simulink model "Nugraha_Setya_Ardi"  (R2020b)
settings: Solver=VariableStepAuto  StartTime=0.0  StopTime=0  RelTol=1e-5
libraries: simulink x6, simulink_extras x5, pid_lib x3, sharedtransform x2, aerolibutil x1, vrlib x1
settings Model: Creator=user  LastModifiedBy=nugra

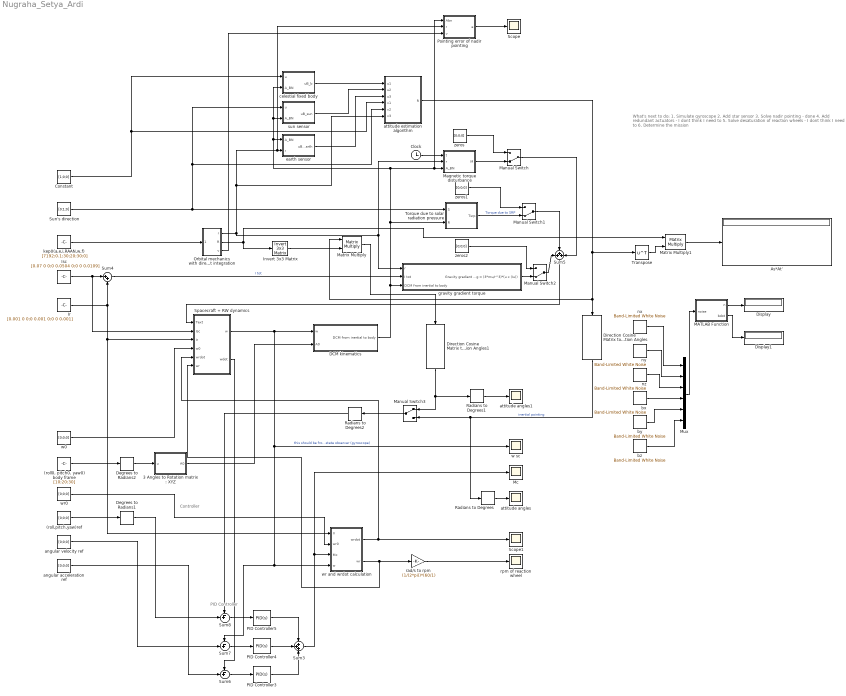
== system Nugraha_Setya_Ardi ==
  note: Controller
  note: PID Controller
  note: What's next to do:
      | 1. Simulate gyroscope
      | 2. Add star sensor
      | 3. Solve nadir pointing - done
      | 4. Add redundant actuators - I dont think I need to
      | 5. Solve desaturation of reaction wheels -  I dont think I need to
      | 6. Determine the mission
  (roll,pitch,yaw)ref : Constant  Value=[0;0;0]  VectorParams1D=off
  "(roll0, pitch0, yaw0) body frame" : Constant  Value=[10;20;30]  VectorParams1D=off
  "3 Angles to Rotation matrix : XYZ" : MATLAB Function  TreatAsAtomicUnit=on
  As*At' : Display
  Clock : Clock
  Constant : Constant  Value=[1;0;0]
  DCM kinematics : Subsystem
  Degrees to Radians1 : simulink_extras/Transformations/Degrees to Radians
  Degrees to Radians2 : simulink_extras/Transformations/Degrees to Radians
  Direction Cosine Matrix to Rotation Angles : sharedtransform/Direction Cosine Matrix to Rotation Angles  rotationOrder=XYZ  aMode=aMode  action=None  tolerance=eps(2)
      settings: SourceProductBaseCode=AE,PW,MT,UV,VE,VP
  Direction Cosine Matrix to Rotation Angles1 : sharedtransform/Direction Cosine Matrix to Rotation Angles  rotationOrder=XYZ  aMode=aMode  action=None  tolerance=eps(2)
      settings: SourceProductBaseCode=AE,PW,MT,UV,VE,VP
  Display : Display
  Display1 : Display
  Invert 3x3 Matrix : aerolibutil/Invert  3x3 Matrix
  Ir : Constant  Value=[0.001 0 0;0 0.001 0;0 0 0.001]  VectorParams1D=off
  Isc : Constant  Value=[0.07 0 0;0 0.0504 0;0 0 0.0109]  VectorParams1D=off
  MATLAB Function : MATLAB Function  TreatAsAtomicUnit=on
  Magnetic torque disturbance : MATLAB Function  TreatAsAtomicUnit=on
  Manual Switch : ManualSwitch  CurrentSetting=0
  Manual Switch1 : ManualSwitch  CurrentSetting=0
  Manual Switch2 : ManualSwitch  CurrentSetting=0
  Manual Switch3 : ManualSwitch
  Matrix Multiply : Product  Multiplication=Matrix(*)
  Matrix Multiply1 : Product  Multiplication=Matrix(*)
  Mc : Scope
  Mux : Mux  Inputs=6
  Orbital mechanics with direct integration : Subsystem
  PID Controller3 : pid_lib/PID Controller  Controller=PID  Form=Parallel  TimeDomain=Continuous-time  UseExternalTs=off  SampleTime=-1  IntegratorMethod=Forward Euler  FilterMethod=Forward Euler  ControllerParametersSource=internal  P=100  I=0  D=0  UseFilter=on  N=100  TunerSelectOption=Transfer Function Based (PID Tuner App)  InitialConditionSource=internal  InitialConditionForIntegrator=0  InitialConditionForFilter=0  DifferentiatorICPrevScaledInput=0  ExternalReset=none  TrackingMode=off  Kt=1  LimitOutput=off  SatLimitsSource=internal  UpperSaturationLimit=inf  LowerSaturationLimit=-inf  LinearizeAsGain=on  AntiWindupMode=none  Kb=1  POutMin=[]  POutMax=[]  IOutMin=[]  IOutMax=[]  DOutMin=[]  DOutMax=[]  NOutMin=[]  NOutMax=[]  SumOutMin=[]  SumOutMax=[]  SaturationOutMin=[]  SaturationOutMax=[]  PParamMin=[]  PParamMax=[]  IParamMin=[]  IParamMax=[]  DParamMin=[]  DParamMax=[]  NParamMin=[]  NParamMax=[]  KbParamMin=[]  KbParamMax=[]  KtParamMin=[]  KtParamMax=[]  KbOutMin=[]  KbOutMax=[]  KtOutMin=[]  KtOutMax=[]  IntegratorOutMin=[]  IntegratorOutMax=[]  FilterOutMin=[]  FilterOutMax=[]  SumI1OutMin=[]  SumI1OutMax=[]  SumI2OutMin=[]  SumI2OutMax=[]  SumI3OutMin=[]  SumI3OutMax=[]  SumI4OutMin=[]  SumI4OutMax=[]  SumDOutMin=[]  SumDOutMax=[]  DifferentiatorOutMin=[]  DifferentiatorOutMax=[]  FilterDiffOutCoefMin=[]  FilterDiffOutCoefMax=[]  ReciprocalOutMin=[]  ReciprocalOutMax=[]  SumDenOutMin=[]  SumDenOutMax=[]  SumNumOutMin=[]  SumNumOutMax=[]  DivideOutMin=[]  DivideOutMax=[]  UdiffTsProdOutMin=[]  UdiffTsProdOutMax=[]  NTsProdOutMin=[]  NTsProdOutMax=[]  UintegralTsProdOutMin=[]  UintegralTsProdOutMax=[]  UngainTsProdOutMin=[]  UngainTsProdOutMax=[]  IntegratorContinuousStateAttributes=''  IntegratorStateMustResolveToSignalObject=off  IntegratorRTWStateStorageClass=Auto  FilterContinuousStateAttributes=''  FilterStateMustResolveToSignalObject=off  FilterRTWStateStorageClass=Auto  ParallelPVariant=InternalParameters  IdealPVariant=Disabled  IVariant=InternalParameters  DVariant=InternalParameters  IntegratorVariant=Continuous  SatVariant=Disabled  AWVariant=Passthrough  PCopyVariant=Disabled  TRVariant=Disabled  FdbkBlocksVariant=Forward  IdealPFdbkVariant=Disabled  SatFdbkVariant=Disabled  DerivativeFilterVariant=ContFilter  NVariant=InternalParameters  NCopyVariant=Disabled  FilterICVariant=InternalICsFilter  IntegratorICVariant=InternalICs  ExternalResetVariant=Disabled  TRSumVariant=Passthrough  SumFdbkVariant=Disabled  SumVariant=Sum_PID  TsampFilterVariant=InternalTs  TsampNgainVariant=Passthrough  TsampIntegralVariant=Passthrough  ExternalSaturationOutDataTypeStr=Inherit: Same as second input
  PID Controller4 : pid_lib/PID Controller  Controller=PID  Form=Parallel  TimeDomain=Continuous-time  UseExternalTs=off  SampleTime=-1  IntegratorMethod=Forward Euler  FilterMethod=Forward Euler  ControllerParametersSource=internal  P=70  I=0  D=0  UseFilter=on  N=100  TunerSelectOption=Transfer Function Based (PID Tuner App)  InitialConditionSource=internal  InitialConditionForIntegrator=0  InitialConditionForFilter=0  DifferentiatorICPrevScaledInput=0  ExternalReset=none  TrackingMode=off  Kt=1  LimitOutput=off  SatLimitsSource=internal  UpperSaturationLimit=inf  LowerSaturationLimit=-inf  LinearizeAsGain=on  AntiWindupMode=none  Kb=1  POutMin=[]  POutMax=[]  IOutMin=[]  IOutMax=[]  DOutMin=[]  DOutMax=[]  NOutMin=[]  NOutMax=[]  SumOutMin=[]  SumOutMax=[]  SaturationOutMin=[]  SaturationOutMax=[]  PParamMin=[]  PParamMax=[]  IParamMin=[]  IParamMax=[]  DParamMin=[]  DParamMax=[]  NParamMin=[]  NParamMax=[]  KbParamMin=[]  KbParamMax=[]  KtParamMin=[]  KtParamMax=[]  KbOutMin=[]  KbOutMax=[]  KtOutMin=[]  KtOutMax=[]  IntegratorOutMin=[]  IntegratorOutMax=[]  FilterOutMin=[]  FilterOutMax=[]  SumI1OutMin=[]  SumI1OutMax=[]  SumI2OutMin=[]  SumI2OutMax=[]  SumI3OutMin=[]  SumI3OutMax=[]  SumI4OutMin=[]  SumI4OutMax=[]  SumDOutMin=[]  SumDOutMax=[]  DifferentiatorOutMin=[]  DifferentiatorOutMax=[]  FilterDiffOutCoefMin=[]  FilterDiffOutCoefMax=[]  ReciprocalOutMin=[]  ReciprocalOutMax=[]  SumDenOutMin=[]  SumDenOutMax=[]  SumNumOutMin=[]  SumNumOutMax=[]  DivideOutMin=[]  DivideOutMax=[]  UdiffTsProdOutMin=[]  UdiffTsProdOutMax=[]  NTsProdOutMin=[]  NTsProdOutMax=[]  UintegralTsProdOutMin=[]  UintegralTsProdOutMax=[]  UngainTsProdOutMin=[]  UngainTsProdOutMax=[]  IntegratorContinuousStateAttributes=''  IntegratorStateMustResolveToSignalObject=off  IntegratorRTWStateStorageClass=Auto  FilterContinuousStateAttributes=''  FilterStateMustResolveToSignalObject=off  FilterRTWStateStorageClass=Auto  ParallelPVariant=InternalParameters  IdealPVariant=Disabled  IVariant=InternalParameters  DVariant=InternalParameters  IntegratorVariant=Continuous  SatVariant=Disabled  AWVariant=Passthrough  PCopyVariant=Disabled  TRVariant=Disabled  FdbkBlocksVariant=Forward  IdealPFdbkVariant=Disabled  SatFdbkVariant=Disabled  DerivativeFilterVariant=ContFilter  NVariant=InternalParameters  NCopyVariant=Disabled  FilterICVariant=InternalICsFilter  IntegratorICVariant=InternalICs  ExternalResetVariant=Disabled  TRSumVariant=Passthrough  SumFdbkVariant=Disabled  SumVariant=Sum_PID  TsampFilterVariant=InternalTs  TsampNgainVariant=Passthrough  TsampIntegralVariant=Passthrough  ExternalSaturationOutDataTypeStr=Inherit: Same as second input
  PID Controller5 : pid_lib/PID Controller  Controller=PID  Form=Parallel  TimeDomain=Continuous-time  UseExternalTs=off  SampleTime=-1  IntegratorMethod=Forward Euler  FilterMethod=Forward Euler  ControllerParametersSource=internal  P=10  I=0  D=0  UseFilter=on  N=100  TunerSelectOption=Transfer Function Based (PID Tuner App)  InitialConditionSource=internal  InitialConditionForIntegrator=0  InitialConditionForFilter=0  DifferentiatorICPrevScaledInput=0  ExternalReset=none  TrackingMode=off  Kt=1  LimitOutput=off  SatLimitsSource=internal  UpperSaturationLimit=inf  LowerSaturationLimit=-inf  LinearizeAsGain=on  AntiWindupMode=none  Kb=1  POutMin=[]  POutMax=[]  IOutMin=[]  IOutMax=[]  DOutMin=[]  DOutMax=[]  NOutMin=[]  NOutMax=[]  SumOutMin=[]  SumOutMax=[]  SaturationOutMin=[]  SaturationOutMax=[]  PParamMin=[]  PParamMax=[]  IParamMin=[]  IParamMax=[]  DParamMin=[]  DParamMax=[]  NParamMin=[]  NParamMax=[]  KbParamMin=[]  KbParamMax=[]  KtParamMin=[]  KtParamMax=[]  KbOutMin=[]  KbOutMax=[]  KtOutMin=[]  KtOutMax=[]  IntegratorOutMin=[]  IntegratorOutMax=[]  FilterOutMin=[]  FilterOutMax=[]  SumI1OutMin=[]  SumI1OutMax=[]  SumI2OutMin=[]  SumI2OutMax=[]  SumI3OutMin=[]  SumI3OutMax=[]  SumI4OutMin=[]  SumI4OutMax=[]  SumDOutMin=[]  SumDOutMax=[]  DifferentiatorOutMin=[]  DifferentiatorOutMax=[]  FilterDiffOutCoefMin=[]  FilterDiffOutCoefMax=[]  ReciprocalOutMin=[]  ReciprocalOutMax=[]  SumDenOutMin=[]  SumDenOutMax=[]  SumNumOutMin=[]  SumNumOutMax=[]  DivideOutMin=[]  DivideOutMax=[]  UdiffTsProdOutMin=[]  UdiffTsProdOutMax=[]  NTsProdOutMin=[]  NTsProdOutMax=[]  UintegralTsProdOutMin=[]  UintegralTsProdOutMax=[]  UngainTsProdOutMin=[]  UngainTsProdOutMax=[]  IntegratorContinuousStateAttributes=''  IntegratorStateMustResolveToSignalObject=off  IntegratorRTWStateStorageClass=Auto  FilterContinuousStateAttributes=''  FilterStateMustResolveToSignalObject=off  FilterRTWStateStorageClass=Auto  ParallelPVariant=InternalParameters  IdealPVariant=Disabled  IVariant=InternalParameters  DVariant=InternalParameters  IntegratorVariant=Continuous  SatVariant=Disabled  AWVariant=Passthrough  PCopyVariant=Disabled  TRVariant=Disabled  FdbkBlocksVariant=Forward  IdealPFdbkVariant=Disabled  SatFdbkVariant=Disabled  DerivativeFilterVariant=ContFilter  NVariant=InternalParameters  NCopyVariant=Disabled  FilterICVariant=InternalICsFilter  IntegratorICVariant=InternalICs  ExternalResetVariant=Disabled  TRSumVariant=Passthrough  SumFdbkVariant=Disabled  SumVariant=Sum_PID  TsampFilterVariant=InternalTs  TsampNgainVariant=Passthrough  TsampIntegralVariant=Passthrough  ExternalSaturationOutDataTypeStr=Inherit: Same as second input
  Pointing error of nadir pointing : MATLAB Function  TreatAsAtomicUnit=on
  Radians to Degrees : simulink_extras/Transformations/Radians to Degrees
  Radians to Degrees1 : simulink_extras/Transformations/Radians to Degrees
  Radians to Degrees2 : simulink_extras/Transformations/Radians to Degrees
  Scope : Scope
  Scope1 : Scope
  Spacecraft + RW dynamics : Subsystem
  Sum3 : Sum  Inputs=+++
  Sum4 : Sum  Inputs=|++
  Sum5 : Sum  Inputs=+++
  Sum6 : Sum  Inputs=-+|
  Sum7 : Sum  Inputs=-+|
  Sum8 : Sum  Inputs=-+|
  Sun's direction : Constant  Value=[0;1;0]
  Torque due to solar radiation pressure : MATLAB Function  TreatAsAtomicUnit=on
  Transpose : Math  Operator=transpose  SaturateOnIntegerOverflow=on
  angular acceleration ref : Constant  Value=[0;0;0]
  angular velocity ref : Constant  Value=[0;0;0]  VectorParams1D=off
  attitude angles : Scope
  attitude angles1 : Scope
  attitude estimation algorithm : MATLAB Function  TreatAsAtomicUnit=on
  bx : simulink/Sources/Band-Limited White Noise  Cov=[0.0001]  Ts=0.001  seed=[236431]
  by : simulink/Sources/Band-Limited White Noise  Cov=[0.0001]  Ts=0.001  seed=[768541]
  bz : simulink/Sources/Band-Limited White Noise  Cov=[0.0001]  Ts=0.001  seed=[287921]
  celestial fixed body : MATLAB Function  TreatAsAtomicUnit=on
  earth sensor : MATLAB Function  TreatAsAtomicUnit=on
  gravity gradient torque : Subsystem
  kep0(a,e,i,RAAN,w,f) : Constant  Value=[7192;0.1;30;20;30;0]  VectorParams1D=off
  nx : simulink/Sources/Band-Limited White Noise  Cov=[0.0001]  Ts=0.01  seed=[23341]
  ny : simulink/Sources/Band-Limited White Noise  Cov=[0.0001]  Ts=0.001  seed=[6341]
  nz : simulink/Sources/Band-Limited White Noise  Cov=[0.0001]  Ts=0.001  seed=[2335671]
  rad/s to rpm : Gain  Gain=(1/(2*pi))*(60/1)
  rpm of reaction wheel : Scope
  sun sensor : MATLAB Function  TreatAsAtomicUnit=on
  w sc : Scope
  w0 : Constant  Value=[0;0;0]
  wr and wrdot calculation : Subsystem
  wr0 : Constant  Value=[0;0;0]
  zeros : Constant  Value=[0;0;0]  VectorParams1D=off
  zeros1 : Constant  Value=[0;0;0]  VectorParams1D=off
  zeros2 : Constant  Value=[0;0;0]  VectorParams1D=off
  wires:
  Isc/1 -> Spacecraft + RW dynamics/2(Isc), Sum4/1
  Ir/1 -> wr and wrdot calculation/1(Ir), Spacecraft + RW dynamics/3(Ir), Sum4/2
  w0/1 -> Spacecraft + RW dynamics/4(w0)
  "(roll0, pitch0, yaw0) body frame"/1 -> Degrees to Radians2/1
  (roll,pitch,yaw)ref/1 -> Degrees to Radians1/1
  angular velocity ref/1 -> Sum7/2
  angular acceleration ref/1 -> Sum6/2
  Degrees to Radians1/1 -> Sum8/2
  Degrees to Radians2/1 -> "3 Angles to Rotation matrix : XYZ"/1(u)
  Torque due to solar radiation pressure/1(Tsrp) -> Manual Switch1/2  "Torque due to SRP"
  Radians to Degrees/1 -> attitude angles/1
  rad/s to rpm/1 -> rpm of reaction wheel/1
  gravity gradient torque/1(Gravity gradient torque Mgg = (3*mu/r^3)*(u x (Iu))) -> Manual Switch2/2
  Sum4/1 -> gravity gradient torque/2(I tot)  "I tot"
  kep0(a,e,i,RAAN,w,f)/1 -> Orbital mechanics with direct integration/1(kep0)
  Sum5/1 -> Spacecraft + RW dynamics/1(Text)
  Spacecraft + RW dynamics/2(wdot) -> Sum6/1
  "3 Angles to Rotation matrix : XYZ"/1(A0) -> DCM kinematics/2(A0)
  wr and wrdot calculation/1(wrdot) -> Spacecraft + RW dynamics/5(wrdot), Scope1/1
  wr and wrdot calculation/2(wr) -> rad/s to rpm/1, Spacecraft + RW dynamics/6(wr)
  wr0/1 -> wr and wrdot calculation/2(wr0)
  Sum6/1 -> PID Controller3/1
  Sum7/1 -> PID Controller4/1
  PID Controller5/1 -> Sum3/1
  PID Controller4/1 -> Sum3/2
  PID Controller3/1 -> Sum3/3
  Sum3/1 -> Mc/1, wr and wrdot calculation/3(Mc)
  Orbital mechanics with direct integration/1(r) -> gravity gradient torque/1(r), Magnetic torque disturbance/2(r), attitude estimation algorithm/6(v3), Pointing error of nadir pointing/2(r), earth sensor/2(r)
  DCM kinematics/1(DCM from inertial to body) -> earth sensor/1(A_BN), celestial fixed body/2(A_BN), sun sensor/2(A_BN), Pointing error of nadir pointing/1(Abn), Magnetic torque disturbance/3(A_BN), Torque due to solar radiation pressure/2(R), gravity gradient torque/3(DCM from inertial to body)
  Clock/1 -> Magnetic torque disturbance/1(t)
  Magnetic torque disturbance/1(M) -> Manual Switch/2
  zeros/1 -> Manual Switch/1
  Manual Switch/1 -> Sum5/3
  zeros1/1 -> Manual Switch1/1
  Manual Switch1/1 -> Sum5/2
  zeros2/1 -> Manual Switch2/1
  Manual Switch2/1 -> Sum5/1
  Sun's direction/1 -> sun sensor/1(u), attitude estimation algorithm/5(v2), Torque due to solar radiation pressure/1(S)
  sun sensor/1(uB_sun) -> attitude estimation algorithm/2(u2)
  earth sensor/1(uB_earth) -> attitude estimation algorithm/3(u3)
  Constant/1 -> celestial fixed body/1(u), attitude estimation algorithm/4(v1)
  celestial fixed body/1(uB_b) -> attitude estimation algorithm/1(u1)
  attitude estimation algorithm/1(R) -> Transpose/1, Matrix Multiply/1, Direction Cosine Matrix to Rotation Angles/1
  Direction Cosine Matrix to Rotation Angles/1 -> Radians to Degrees/1, Manual Switch3/2  "inertial pointing"
  Spacecraft + RW dynamics/1(w) -> Sum7/1, wr and wrdot calculation/4(w), w sc/1, DCM kinematics/1(w)  "this should be from state observer (gyroscope)"
  Orbital mechanics with direct integration/2(R) -> Invert 3x3 Matrix/1, Matrix Multiply1/1
  Sum8/1 -> PID Controller5/1
  Invert 3x3 Matrix/1 -> Matrix Multiply/2
  Matrix Multiply/1 -> Direction Cosine Matrix to Rotation Angles1/1
  Manual Switch3/1 -> Radians to Degrees2/1
  Direction Cosine Matrix to Rotation Angles1/1 -> Radians to Degrees1/1, Manual Switch3/1
  Radians to Degrees1/1 -> attitude angles1/1
  Transpose/1 -> Matrix Multiply1/2
  Matrix Multiply1/1 -> As*At'/1
  Pointing error of nadir pointing/1(e) -> Scope/1
  Orbital mechanics with direct integration/3(v) -> Pointing error of nadir pointing/3(v)
  Radians to Degrees2/1 -> Sum8/1
  MATLAB Function/1(n) -> Display/1
  MATLAB Function/2(bdot) -> Display1/1
  nx/1 -> Mux/1
  ny/1 -> Mux/2
  nz/1 -> Mux/3
  bx/1 -> Mux/4
  by/1 -> Mux/5
  bz/1 -> Mux/6
  Mux/1 -> MATLAB Function/1(noise)

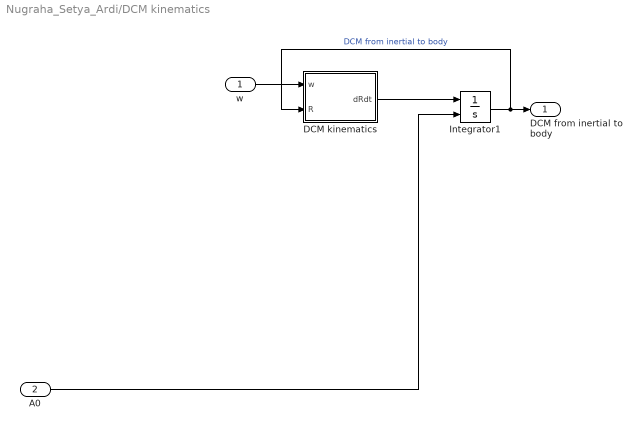
== system Nugraha_Setya_Ardi/DCM kinematics ==
  w : Inport
  A0 : Inport  Port=2
  DCM kinematics : MATLAB Function  TreatAsAtomicUnit=on
  Integrator1 : Integrator  InitialConditionSource=external
  DCM from inertial to body : Outport
  wires:
  DCM kinematics/1(dRdt) -> Integrator1/1
  A0/1 -> Integrator1/2
  Integrator1/1 -> DCM kinematics/2(R), DCM from inertial to body/1  "DCM from inertial to body"
  w/1 -> DCM kinematics/1(w)

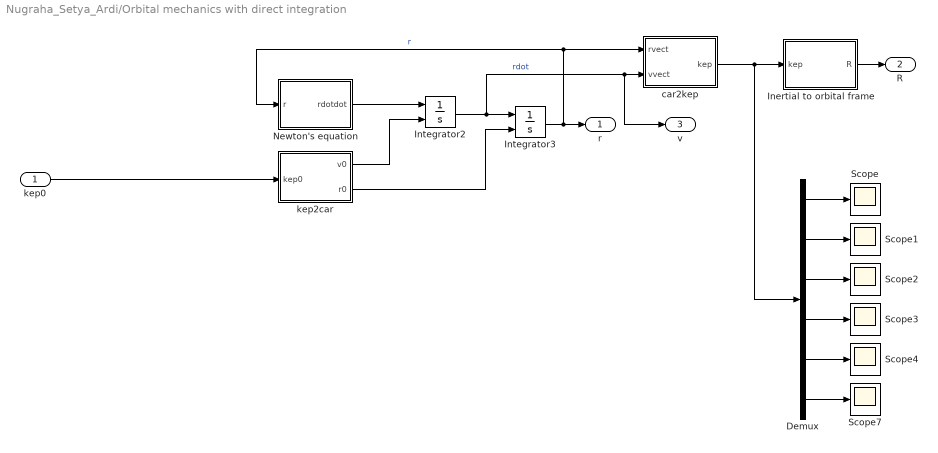
== system Nugraha_Setya_Ardi/Orbital mechanics with direct integration ==
  kep0 : Inport
  Demux : Demux  Outputs=6
  Inertial to orbital frame : MATLAB Function  TreatAsAtomicUnit=on
  Integrator2 : Integrator  InitialConditionSource=external
  Integrator3 : Integrator  InitialConditionSource=external
  Newton's equation : MATLAB Function  TreatAsAtomicUnit=on
  Scope{,1..4,7} (6 alike) : Scope
  car2kep : MATLAB Function  TreatAsAtomicUnit=on
  kep2car : MATLAB Function  TreatAsAtomicUnit=on
  r : Outport
  R : Outport  Port=2
  v : Outport  Port=3
  wires:
  Integrator3/1 -> car2kep/1(rvect), Newton's equation/1(r), r/1  "r"
  Newton's equation/1(rdotdot) -> Integrator2/1
  kep2car/2(r0) -> Integrator3/2
  kep2car/1(v0) -> Integrator2/2
  kep0/1 -> kep2car/1(kep0)
  Integrator2/1 -> v/1, car2kep/2(vvect), Integrator3/1  "rdot"
  car2kep/1(kep) -> Demux/1, Inertial to orbital frame/1(kep)
  Inertial to orbital frame/1(R) -> R/1
  Demux/1 -> Scope/1
  Demux/2 -> Scope1/1
  Demux/3 -> Scope2/1
  Demux/4 -> Scope3/1
  Demux/5 -> Scope4/1
  Demux/6 -> Scope7/1

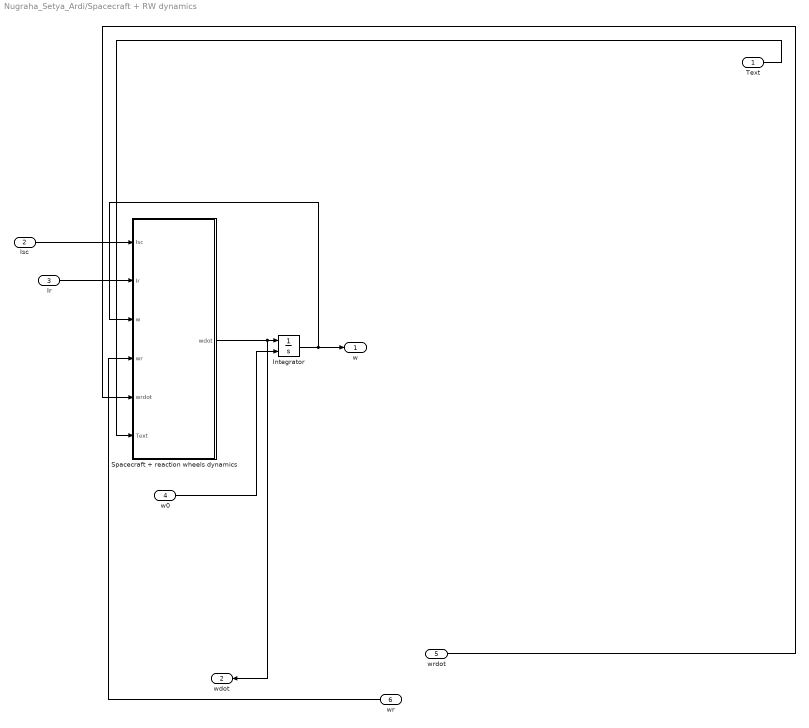
== system Nugraha_Setya_Ardi/Spacecraft + RW dynamics ==
  Text : Inport
  Isc : Inport  Port=2
  Ir : Inport  Port=3
  w0 : Inport  Port=4
  wrdot : Inport  Port=5
  wr : Inport  Port=6
  Integrator : Integrator  InitialConditionSource=external
  Spacecraft + reaction wheels dynamics : MATLAB Function  TreatAsAtomicUnit=on
  w : Outport
  wdot : Outport  Port=2
  wires:
  Text/1 -> Spacecraft + reaction wheels dynamics/6(Text)
  w0/1 -> Integrator/2
  Spacecraft + reaction wheels dynamics/1(wdot) -> wdot/1, Integrator/1
  Isc/1 -> Spacecraft + reaction wheels dynamics/1(Isc)
  wr/1 -> Spacecraft + reaction wheels dynamics/4(wr)
  wrdot/1 -> Spacecraft + reaction wheels dynamics/5(wrdot)
  Integrator/1 -> Spacecraft + reaction wheels dynamics/3(w), w/1
  Ir/1 -> Spacecraft + reaction wheels dynamics/2(Ir)

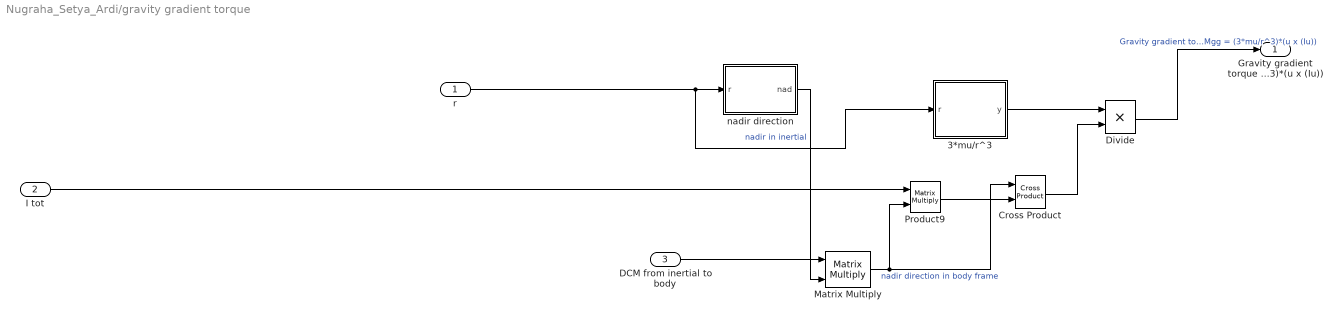
== system Nugraha_Setya_Ardi/gravity gradient torque ==
  r : Inport
  I tot : Inport  Port=2
  DCM from inertial to body : Inport  Port=3
  3*mu/r^3 : MATLAB Function  TreatAsAtomicUnit=on
  Cross Product : vrlib/Utilities/Cross Product
  Divide : Product  Inputs=**
  Matrix Multiply : Product  Multiplication=Matrix(*)
  Product9 : Product  Multiplication=Matrix(*)
  nadir direction : MATLAB Function  TreatAsAtomicUnit=on
  Gravity gradient torque Mgg = (3*mu/r^3)*(u x (Iu)) : Outport
  wires:
  Matrix Multiply/1 -> Product9/2, Cross Product/1  "nadir direction in body frame"
  Divide/1 -> Gravity gradient torque Mgg = (3*mu/r^3)*(u x (Iu))/1  "Gravity gradient torque Mgg = (3*mu/r^3)*(u x (Iu))"
  3*mu/r^3/1(y) -> Divide/1
  nadir direction/1(nad) -> Matrix Multiply/2  "nadir in inertial"
  DCM from inertial to body/1 -> Matrix Multiply/1
  I tot/1 -> Product9/1
  r/1 -> 3*mu/r^3/1(r), nadir direction/1(r)
  Product9/1 -> Cross Product/2
  Cross Product/1 -> Divide/2

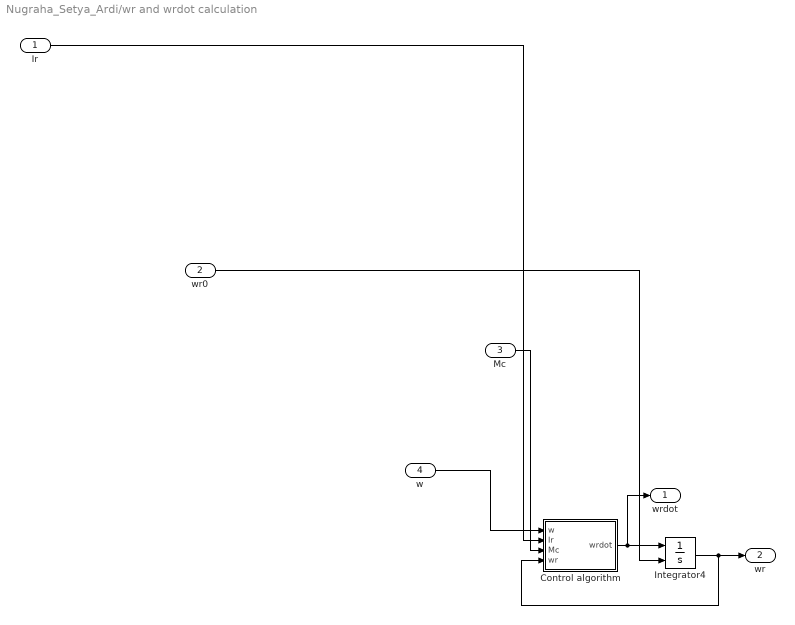
== system Nugraha_Setya_Ardi/wr and wrdot calculation ==
  Ir : Inport
  wr0 : Inport  Port=2
  Mc : Inport  Port=3
  w : Inport  Port=4
  Control algorithm : MATLAB Function  TreatAsAtomicUnit=on
  Integrator4 : Integrator  InitialConditionSource=external
  wrdot : Outport
  wr : Outport  Port=2
  wires:
  Control algorithm/1(wrdot) -> wrdot/1, Integrator4/1
  Ir/1 -> Control algorithm/2(Ir)
  wr0/1 -> Integrator4/2
  Mc/1 -> Control algorithm/3(Mc)
  w/1 -> Control algorithm/1(w)
  Integrator4/1 -> Control algorithm/4(wr), wr/1

== matlab function Nugraha_Setya_Ardi/earth sensor ==
  data: A_BN input; uB_earth output; r input
function uB_earth = fcn(A_BN,r)
rdir = -r/norm(r);
uB_earth = A_BN*rdir

== matlab function Nugraha_Setya_Ardi/celestial fixed body ==
  data: u input; uB_b output; A_BN input
function uB_b = fcn(u,A_BN)
udir = u/norm(u);
uB_b = A_BN*udir

== matlab function Nugraha_Setya_Ardi/attitude estimation algorithm ==
  data: u1 input; R output; u2 input; u3 input; v1 input; v2 input; v3 input
function R = fcn(u1,u2,u3,v1,v2,v3)
% Analytic Solution to Wahba's Problem
v3dir = -v3/norm(v3);
B1 = u1*v1';
B2 = u2*v2';
B3 = u3*v3dir';
B = B1+B2+B3;
[U,S,V]=svd(B);
R = U*[1 0 0;0 1 0;0 0 det(U)*det(V)]*V';

== matlab function Nugraha_Setya_Ardi/Orbital mechanics with direct integration/car2kep ==
  data: rvect input; kep output; vvect input
function kep = fcn(rvect,vvect)
mu = astroConstants(13);
r = norm(rvect);
v = norm(vvect)
a = (mu/2)*(mu/r-v^2/2)^-1;
hvect = cross(rvect,vvect);
h = norm(hvect);
k = [0;0;1];
i = acos(dot(hvect,k)/h);
Nhat = cross(k,hvect)/norm(cross(k,hvect));
if Nhat(2,1) >=0
    Om = acos(Nhat(1,1));
else
    Om = 2*pi - acos(Nhat(1,1));
end

evect = cross(vvect,hvect)/mu - rvect/norm(rvect);
e = norm(evect);

%if evect(3,1) >= 0
    w = acos(dot(Nhat,evect/e));
% else
%     w = 2*pi-acos(dot(Nhat,evect/e));
% end

if dot(vvect,rvect) >= 0
    theta = acos(dot(evect/e,rvect/norm(rvect)));
else
    theta = 2*pi - acos(dot(evect/e,rvect/norm(rvect)));
end
kep = [a;e;rad2deg(i);rad2deg(Om);rad2deg(w);rad2deg(theta)];

== matlab function Nugraha_Setya_Ardi/Orbital mechanics with direct integration/Inertial to orbital frame ==
  data: kep input; R output
function R = fcn(kep)
a = kep(1,1);
e = kep(2,1);
i = deg2rad(kep(3,1));
RA = deg2rad(kep(4,1));
w = deg2rad(kep(5,1));
f = deg2rad(kep(6,1));

R3_W = [ cos(RA) sin(RA) 0; -sin(RA) cos(RA) 0; 0 0 1];
R1_i= [1 0 0; 0 cos(i) sin(i); 0 -sin(i) cos(i)];
R3_w = [ cos(w) sin(w) 0; -sin(w) cos(w) 0; 0 0 1];
R3_f = [ cos(f) sin(f) 0; -sin(f) cos(f) 0; 0 0 1];
R3_pi = [ cos(pi) sin(pi) 0; -sin(pi) cos(pi) 0; 0 0 1];
R = R3_pi*R3_f*R3_w*R1_i*R3_W;

== matlab function Nugraha_Setya_Ardi/Pointing error of nadir pointing ==
  data: Abn input; r input; e output; v input
function e = fcn(Abn,r,v)
xb = [1;0;0];
yb = [0;1;0];
zb = [0;0;1];
z = cross(r,v);
y = cross(z,r);
xdir = Abn*(-r/norm(r));
ydir = Abn*(-y/norm(y));
zdir = Abn*(z/norm(z));
ex = rad2deg(acos(dot(xb,xdir)/(norm(xb)*norm(xdir))));
ey = rad2deg(acos(dot(yb,ydir)/(norm(yb)*norm(ydir))));
ez = rad2deg(acos(dot(zb,zdir)/(norm(zb)*norm(zdir))));
e = [ex ey ez]

== matlab function Nugraha_Setya_Ardi/DCM kinematics/DCM kinematics ==
  data: w input; dRdt output; R input
function dRdt = fcn(w,R)
w1 = w(1,1);
w2 = w(2,1);
w3 = w(3,1);
wmat = [0 w3 -w2;-w3 0 w1;w2 -w1 0];
dRdt = wmat*R

== matlab function Nugraha_Setya_Ardi/MATLAB Function ==
  data: n output; bdot output; noise input
function [n,bdot] = fcn(noise)
nx = noise(1);
ny = noise(2);
nz = noise(3);
bx = noise(4);
by = noise(5);
bz = noise(6);
ARW = 0.15;
RRW = 0.0003;
sn = (0.15/sqrt(3600/262))*pi/180;
sb = (0.0003/sqrt(3600/262))*pi/180;
n = sn*[nx;ny;nz];
bdot = sb*[bx;by;bz];

== matlab function Nugraha_Setya_Ardi/Spacecraft + RW dynamics/Spacecraft + reaction wheels dynamics ==
  data: Isc input; wdot output; Ir input; w input; wr input; wrdot input; Text input
function wdot = fcn(Isc,Ir,w,wr,wrdot,Text)
wdot = inv(Isc)*(Text - cross(w,(Isc*w)) + Ir*wrdot + cross(w,(Ir*wr)));

== matlab function Nugraha_Setya_Ardi/Orbital mechanics with direct integration/Newton's equation ==
  data: r input; rdotdot output
function rdotdot = fcn(r)
mu = 3.98600433e+5;
rnorm = norm(r)
rdotdot = (-mu/rnorm^3)*r

== matlab function Nugraha_Setya_Ardi/wr and wrdot calculation/Control algorithm ==
  data: w input; Ir input; Mc input; wrdot output; wr input
function wrdot = fcn(w,Ir,Mc,wr)
wrdot = inv(Ir)*(-Mc-cross(w,(Ir*wr)));

== matlab function Nugraha_Setya_Ardi/gravity gradient torque/nadir direction ==
  data: r input; nad output
function nad = fcn(r)
nad = -r/norm(r)

== matlab function Nugraha_Setya_Ardi/3 Angles to Rotation matrix : XYZ ==
  data: u input; A0 output
function A0 = fcn(u)
ph = u(1,1);
t = u(2,1);
ps = u(3,1);

a11 = cos(ps)*cos(t);
a12 = cos(ps)*sin(t)*sin(ph)+sin(ps)*cos(ph);
a13 = -cos(ps)*sin(t)*cos(ph)+sin(ps)*sin(ph);
a21 = -sin(ps)*cos(t);
a22 = -sin(ps)*sin(t)*sin(ph)+cos(ps)*cos(ph);
a23 = sin(ps)*sin(t)*cos(ph)+cos(ps)*sin(ph);
a31 = sin(t);
a32 = -cos(t)*sin(ph);
a33 = cos(t)*cos(ph);
A0 = [a11 a12 a13;a21 a22 a23;a31 a32 a33];

== matlab function Nugraha_Setya_Ardi/Orbital mechanics with direct integration/kep2car ==
  data: v0 output; kep0 input; r0 output
function [v0,r0] = fcn(kep0)
mu = 3.98600433e+5
a = kep0(1,1);
e = kep0(2,1);
i = deg2rad(kep0(3,1));
RA = deg2rad(kep0(4,1));
w = deg2rad(kep0(5,1));
f = deg2rad(kep0(6,1));

h=sqrt(mu*a*(1-e^2));
rp = (h^2/mu) * (1/(1 + e*cos(f))) * (cos(f)*[1;0;0] + sin(f)*[0;1;0]);
vp = (mu/h) * (-sin(f)*[1;0;0] + (e + cos(f))*[0;1;0]);

R3_W = [ cos(RA) sin(RA) 0; -sin(RA) cos(RA) 0; 0 0 1];
R1_i= [1 0 0; 0 cos(i) sin(i); 0 -sin(i) cos(i)];
R3_w = [ cos(w) sin(w) 0; -sin(w) cos(w) 0; 0 0 1];

Q_pX = (R3_w*R1_i*R3_W);

r = Q_pX'*rp;
v = Q_pX'*vp;
% Convert r and v into row vectors:
r0 = r;
v0 = v;

== matlab function Nugraha_Setya_Ardi/gravity gradient torque/3*mu//r^3 ==
  data: r input; y output
function y = fcn(r)
mu = astroConstants(13);
y= 3*mu/norm(r)^3;

== matlab function Nugraha_Setya_Ardi/Magnetic torque disturbance ==
  data: t input; r input; M output; A_BN input
function M  = fcn(t,r,A_BN)
rhat = r/norm(r);
R = 6371;
w = 2*pi/(24*3600);
% IGRF 1995
g10 = -29682*10^-9;
g11 = -1789*10^-9;
h11 = 5318*10^-9;
H0 = (g10^2 + g11^2 + h11^2)^0.5;
mhat = [sin(deg2rad(11.5))*cos(w*t);sin(deg2rad(11.5))*sin(w*t);cos(deg2rad(11.5))]
bN = (H0*R^3/norm(r)^3)*(3*dot(mhat,rhat)*rhat-mhat);
bB = A_BN*bN;
m = [0.01;0.05;0.01];
M = cross(m,bB);

== matlab function Nugraha_Setya_Ardi/Torque due to solar radiation pressure ==
  data: S input; R input; Tsrp output
function Tsrp   = fcn(S,R)
% deviation of centre of mass from geometric center
% Spacecraft main body
n1 = [1;0;0];
A1 = 0.3*0.3;
n2 = [0;1;0];
A2 = 0.3*0.8;
n3 = [0;0;1];
A3 = 0.3*0.8;
n4 = -n1;
A4 = A1;
n5 = -n2;
A5 = A2;
n6 = -n3;
A6 = A3;
rhoS1 = 0.5;
rhoD1 = 0.1;

% Solar panel
n7 = [0;0;1];
A7 = 0.3*1;
n8 = -n7;
A8 = A7;
n9 = [0;0;1];
A9 = A7;
n10 = -n9;
A10 = A7;
rhoS2 = 0.8;
rhoD2 = 0.1;

%defined
SB = (R*S)/(norm(R*S));
P = 1358/299792458;
d1 = dot(SB,n1);
d2 = dot(SB,n2);
d3 = dot(SB,n3);
d4 = dot(SB,n4);
d5 = dot(SB,n5);
d6 = dot(SB,n6);
d7 = dot(SB,n7);
d8 = dot(SB,n8);
d9 = dot(SB,n9);
d10 = dot(SB,n10);
%fx = -P*A1*d1*((1-rhoS1)*SB+(2*rhoS1*d1+(2/3)*rhoD1)*n1);
%face 1
if d1 < 0
    f1 =  [0;0;0];
else
    f1 = -P*A1*d1*((1-rhoS1)*SB+(2*rhoS1*d1+(2/3)*rhoD1)*n1);
end

%face2
if d2 < 0
    f2 =  [0;0;0];
else
    f2 = -P*A2*d2*((1-rhoS1)*SB+(2*rhoS1*d2+(2/3)*rhoD1)*n2);
end

% face 3
if d3 < 0
    f3 =  [0;0;0];
else
    f3 = -P*A3*d3*((1-rhoS1)*SB+(2*rhoS1*d3+(2/3)*rhoD1)*n3);
end

%face 4
if d4 < 0
    f4 =  [0;0;0];
else
    f4 = -P*A4*d4*((1-rhoS1)*SB+(2*rhoS1*d4+(2/3)*rhoD1)*n4);
end

%face 5
if d5 < 0
    f5 =  [0;0;0];
else
    f5 = -P*A5*d5*((1-rhoS1)*SB+(2*rhoS1*d5+(2/3)*rhoD1)*n5);
end

%face 6
if d6 < 0
    f6 =  [0;0;0];
else
    f6 = -P*A6*d6*((1-rhoS1)*SB+(2*rhoS1*d6+(2/3)*rhoD1)*n6);
end

% face 7
if d7 < 0
    f7 =  [0;0;0];
else
    f7 = -P*A7*d7*((1-rhoS2)*SB+(2*rhoS2*d7+(2/3)*rhoD2)*n7);
end

% face 8
if d8 < 0
    f8 =  [0;0;0];
else
    f8 = -P*A8*d8*((1-rhoS2)*SB+(2*rhoS2*d8+(2/3)*rhoD2)*n8);
end

% face 9
if d9 < 0
    f9 =  [0;0;0];
else
    f9 = -P*A9*d9*((1-rhoS2)*SB+(2*rhoS2*d9+(2/3)*rhoD2)*n9);
end

% face 10
if d10 < 0
    f10 =  [0;0;0];
else
    f10 = -P*A10*d10*((1-rhoS2)*SB+(2*rhoS2*d10+(2/3)*rhoD2)*n10);
end

r7 = [-0.1;-0.5;0];
r8 = r7;
r9 = [-0.1;0.5;0];
r10 = r9;
f = f8;
Tsrp = cross(r7,f7) + cross(r8,f8) + cross(r9,f9) + cross(r10,f10);
x1 = cross(r7,f7)
x2 = cross(r8,f8)
x3 = cross(r9,f9)
x4 = cross(r10,f10)

== matlab function Nugraha_Setya_Ardi/sun sensor ==
  data: u input; uB_sun output; A_BN input
function uB_sun = fcn(u,A_BN)
udir = u/norm(u);
uB_sun = A_BN*udir;
